simulink model "YFOULIS_LQR_INTEGRATOR"  (R2020a)
settings: Solver=VariableStepAuto  StartTime=0.0  StopTime=10.0  RelTol=1e-3
values from neighbouring files (symbols this model uses):
  K = lqr(sys.A,sys.B,Q,R)    [LQGControl.m]    (also in LQRControl.m; LQRcontrol_with_Integrator.m; MPC.m = 0.028)
  sys = ss(A,B,C,D)    [Blocks_LQR.m]    (also in Blocks_LQRbasic.m; MPC.m = ss(a,b,c,d))
  x0 = zeros(12,1)    [Blocks_LQR.m]    (also in LQGControl.m; LQRControl.m; LQRcontrol_with_Integrator.m; animation_LQG.m = 10)
undefined symbols (not defined in the file or in its folder): Kz
settings Model: Creator=Xrisostomos  LastModifiedBy=Xrisostomos

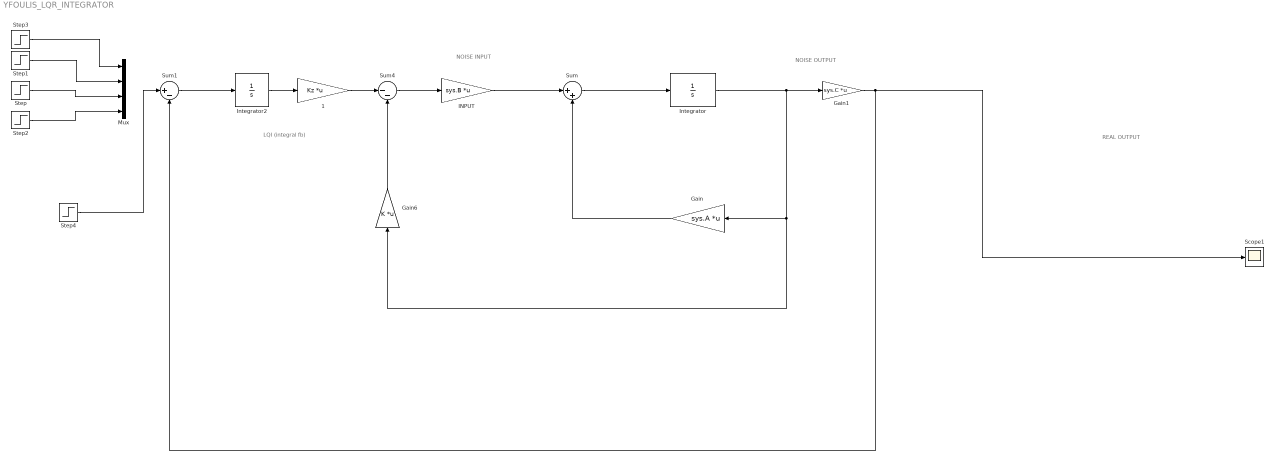
== system YFOULIS_LQR_INTEGRATOR ==
  note: NOISE OUTPUT
  note: REAL OUTPUT
  note: NOISE INPUT
  note: LQI
      | (integral fb)
  1 : Gain  Gain=Kz  Multiplication=Matrix(K*u)
  Gain : Gain  Gain=sys.A  Multiplication=Matrix(K*u)
  Gain1 : Gain  Gain=sys.C  Multiplication=Matrix(K*u)
  Gain6 : Gain  Gain=K  Multiplication=Matrix(K*u)
  INPUT : Gain  Gain=sys.B  Multiplication=Matrix(K*u)
  Integrator : Integrator  InitialCondition=x0
  Integrator2 : Integrator  InitialCondition=x0
  Mux : Mux
  Scope1 : Scope
  Step{,1..4} (5 alike) : Step  SampleTime=0
  Sum : Sum  Inputs=|++
  Sum1 : Sum  Inputs=|+-
  Sum4 : Sum  Inputs=|--
  wires:
  Integrator/1 -> Gain1/1, Gain6/1, Gain/1
  1/1 -> Sum4/1
  Sum4/1 -> INPUT/1
  Step/1 -> Mux/3
  Step2/1 -> Mux/4
  Integrator2/1 -> 1/1
  Gain6/1 -> Sum4/2
  Step1/1 -> Mux/2
  Sum/1 -> Integrator/1
  INPUT/1 -> Sum/1
  Gain/1 -> Sum/2
  Gain1/1 -> Scope1/1, Sum1/2
  Step3/1 -> Mux/1
  Sum1/1 -> Integrator2/1
  Step4/1 -> Sum1/1
